simulink model "HPF"  (R2020b)
settings: Solver=VariableStepAuto  StartTime=0.0  StopTime=10.0  RelTol=1e-3
settings Model: Creator=com  LastModifiedBy=com

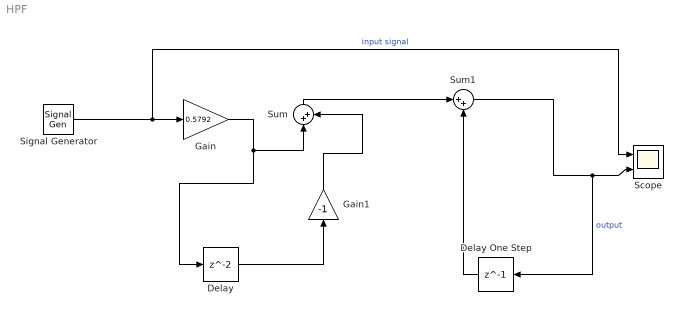
== system HPF ==
  Delay : Delay
  Delay One Step : Delay  DelayLength=1
  Gain : Gain  Gain=0.5792
  Gain1 : Gain  Gain=-1
  Scope : Scope  NumInputPorts=2
  Signal Generator : SignalGenerator  Units=rad/sec
  Sum : Sum  Inputs=|++
  Sum1 : Sum  Inputs=|++
  wires:
  Sum/1 -> Sum1/1
  Sum1/1 -> Delay One Step/1, Scope/2  "output"
  Delay One Step/1 -> Sum1/2
  Gain1/1 -> Sum/2
  Gain/1 -> Sum/1, Delay/1
  Signal Generator/1 -> Scope/1, Gain/1  "input signal"
  Delay/1 -> Gain1/1
